simulink subsystem "tehrani_alv_mass_balance_co2_v3"  (R2019b)
settings: Solver=VariableStepAuto  StartTime=0.0  StopTime=10.0  RelTol=1e-3
settings Model: Creator=RH  LastModifiedBy=RH

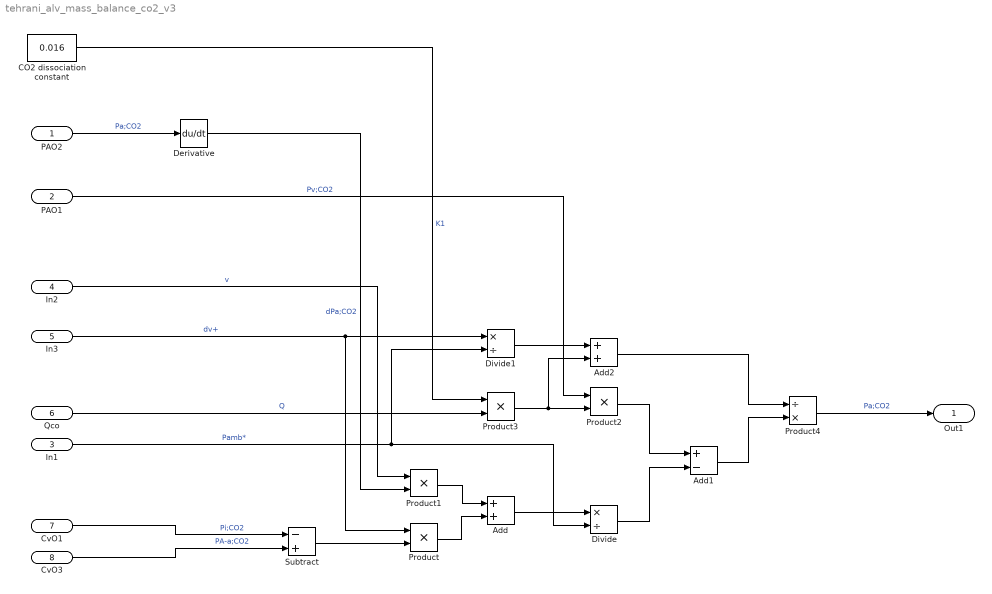
== system tehrani_alv_mass_balance_co2_v3 ==
  PAO2 : Inport
  PAO1 : Inport  Port=2
  In1 : Inport  Port=3
  In2 : Inport  Port=4
  In3 : Inport  Port=5
  Qco : Inport  Port=6
  CvO1 : Inport  Port=7
  CvO3 : Inport  Port=8
  Add : Sum
  Add1 : Sum  Inputs=+-
  Add2 : Sum
  CO2 dissociation constant : Constant  Value=0.016
  Derivative : Derivative
  Divide : Product  Inputs=*/
  Divide1 : Product  Inputs=*/
  Product{,1..3} (4 alike) : Product
  Product4 : Product  Inputs=/*
  Subtract : Sum  Inputs=-+
  Out1 : Outport
  wires:
  In3/1 -> Divide1/1, Product/1  "dv+"
  Add/1 -> Divide/1
  Product1/1 -> Add/1
  In2/1 -> Product1/1  "v"
  Product/1 -> Add/2
  PAO2/1 -> Derivative/1  "Pa;CO2"
  CvO3/1 -> Subtract/2  "PA-a;CO2"
  In1/1 -> Divide1/2, Divide/2  "Pamb*"
  CvO1/1 -> Subtract/1  "Pi;CO2"
  Derivative/1 -> Product1/2  "dPa;CO2"
  Product4/1 -> Out1/1  "Pa;CO2"
  Subtract/1 -> Product/2
  Qco/1 -> Product3/2  "Q"
  PAO1/1 -> Product2/1  "Pv;CO2"
  CO2 dissociation constant/1 -> Product3/1  "K1"
  Product2/1 -> Add1/1
  Divide/1 -> Add1/2
  Product3/1 -> Product2/2, Add2/2
  Divide1/1 -> Add2/1
  Add2/1 -> Product4/1
  Add1/1 -> Product4/2
